simulink model "encode_decode_withAlarms"  (R2022b)
settings: Solver=VariableStepAuto  StartTime=0.0  StopTime=160  RelTol=1e-3
libraries: simulink x8, spsSampleandHoldLib x3
settings Model: Creator=mluser  LastModifiedBy=mluser

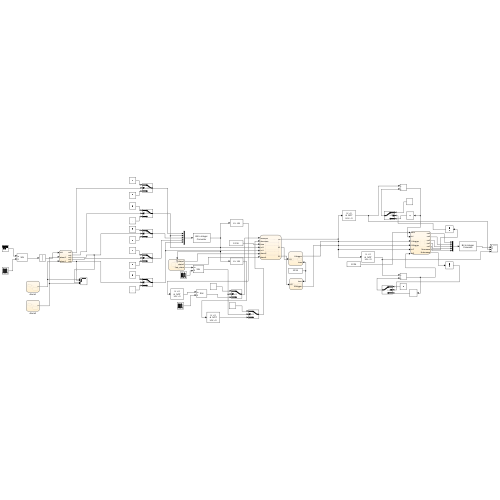
[thumbnail: Simulink's stored preview of the top-level diagram]
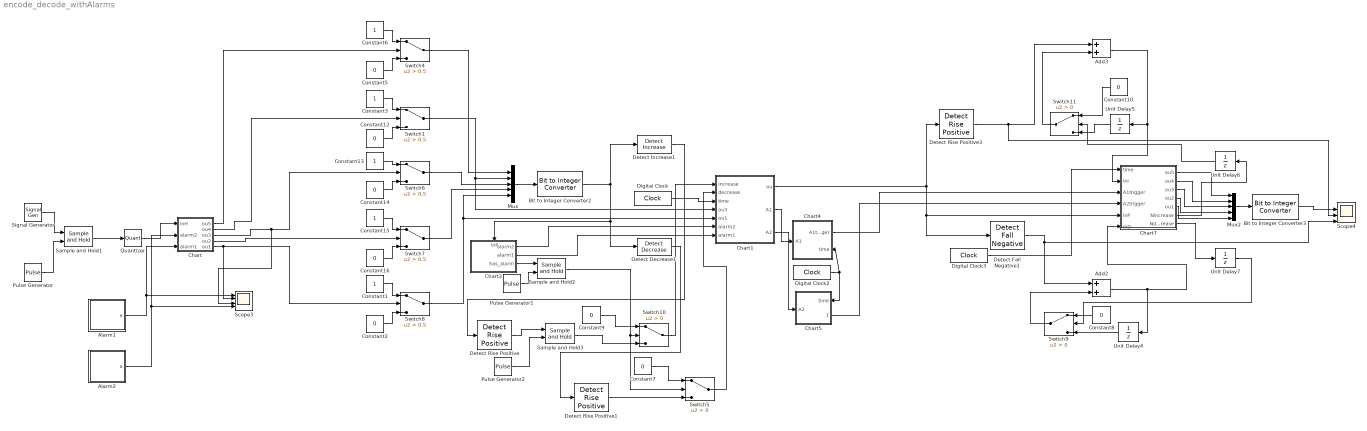
== system encode_decode_withAlarms ==
  Add2 : Sum
  Add3 : Sum
  Alarm1 : Stateflow chart  TreatAsAtomicUnit=on
  Alarm2 : Stateflow chart  TreatAsAtomicUnit=on
  Bit to Integer Converter2 : simulink/Logic and Bit Operations/Bit to Integer Converter  nbits=5  bitOrder=MSB first  signedOutputValues=Unsigned  outDtype=Inherit via internal rule  outDtypeSigned=Inherit via internal rule
      settings: LibrarySourceBlock=|
      | commutil2/Bit to Integer
      | Converter
  Bit to Integer Converter3 : simulink/Logic and Bit Operations/Bit to Integer Converter  nbits=5  bitOrder=MSB first  signedOutputValues=Unsigned  outDtype=Inherit via internal rule  outDtypeSigned=Inherit via internal rule
      settings: LibrarySourceBlock=|
      | commutil2/Bit to Integer
      | Converter
  Chart : Stateflow chart  TreatAsAtomicUnit=on
      settings: PortSchema="{\"entries\":[{\"content\":{\"sides\":[{\"content\":{\"connectorIds\":[\"In1\",\"In2\",\"In3\"]},\"type\":\"ConnectorPlacement.EquallySpacedRectSide\",\"uuid\":\"aaeedc4a-65ef-4d8f-ba01-1ddc4e011816\"},{\"content\":{\"connectorIds\":[\"Out5\",\"Out2\",\"Out1\",\"Out3\",\"Out4\"],\"side\":\"RIGHT\"},\"type\":\"ConnectorPlacement.EquallySpacedRectSide\",\"uuid\":\"bfc75945-f598-4b29-99c0-df6bb3f156b5\"},{\"content\":{\"connectorIds\":[],\"side\":\"TOP\"},\"type\":\"ConnectorPlacement.EquallySpacedRectSide\",\"uuid\":\"e78d9c07-753c-4a5b-aa63-095c584c660c\"}]},\"type\":\"ConnectorPlacement.EquallySpacedConnector\",\"uuid\":\"f46ef6be-e67f-4bb7-838b-d108f8d3e6f5\"}],\"packageUris\":[\"http://schema.mathworks.com/mf0/Connector/R2020b\"],\"version\":\"1.0\"}"
  Chart1 : Stateflow chart  TreatAsAtomicUnit=on
  Chart3 : Stateflow chart  TreatAsAtomicUnit=on
      settings: PortSchema="{\"entries\":[{\"content\":{\"sides\":[{\"content\":{\"connectorIds\":[]},\"type\":\"ConnectorPlacement.EquallySpacedRectSide\",\"uuid\":\"5c3dd9c4-40fc-475e-8fc4-53a3db762fc4\"},{\"content\":{\"connectorIds\":[\"Out1\",\"Out2\",\"Out3\"],\"side\":\"RIGHT\"},\"type\":\"ConnectorPlacement.EquallySpacedRectSide\",\"uuid\":\"288f4f63-e8ff-4ace-a90f-863d45689e1d\"},{\"content\":{\"connectorIds\":[\"In1\"],\"side\":\"TOP\"},\"type\":\"ConnectorPlacement.EquallySpacedRectSide\",\"uuid\":\"c4c1c7c7-df9c-4060-9033-81f7d31c6bbf\"}]},\"type\":\"ConnectorPlacement.EquallySpacedConnector\",\"uuid\":\"fd27b28a-c6e9-46f2-af96-6d8beda93238\"}],\"packageUris\":[\"http://schema.mathworks.com/mf0/Connector/R2020b\"],\"version\":\"1.0\"}"
  Chart4 : Stateflow chart  TreatAsAtomicUnit=on
      settings: PortSchema="{\"entries\":[{\"content\":{\"sides\":[{\"content\":{\"connectorIds\":[\"In2\"]},\"type\":\"ConnectorPlacement.EquallySpacedRectSide\",\"uuid\":\"446bd760-2446-4d27-a1b4-b9f2637686cc\"},{\"content\":{\"connectorIds\":[\"Out1\",\"In1\"],\"side\":\"RIGHT\"},\"type\":\"ConnectorPlacement.EquallySpacedRectSide\",\"uuid\":\"31dc2807-aea3-41af-817a-dc746d332e0b\"},{\"content\":{\"connectorIds\":[],\"side\":\"TOP\"},\"type\":\"ConnectorPlacement.EquallySpacedRectSide\",\"uuid\":\"1029dd63-400c-467c-987d-c8090033263d\"},{\"content\":{\"connectorIds\":[],\"side\":\"BOTTOM\"},\"type\":\"ConnectorPlacement.EquallySpacedRectSide\",\"uuid\":\"3be6e891-aee5-42f4-8a4a-273d783635a4\"}]},\"type\":\"ConnectorPlacement.EquallySpacedConnector\",\"uuid\":\"838269c8-6f3e-4b67-b3d3-f8aaab74d030\"}],\"packageUris\":[\"http://schema.mathworks.com/mf0/Connector/R2020b\"],\"version\":\"1.0\"}"
  Chart5 : Stateflow chart  TreatAsAtomicUnit=on
      settings: PortSchema="{\"entries\":[{\"content\":{\"sides\":[{\"content\":{\"connectorIds\":[\"In2\"]},\"type\":\"ConnectorPlacement.EquallySpacedRectSide\",\"uuid\":\"446bd760-2446-4d27-a1b4-b9f2637686cc\"},{\"content\":{\"connectorIds\":[\"In1\",\"Out1\"],\"side\":\"RIGHT\"},\"type\":\"ConnectorPlacement.EquallySpacedRectSide\",\"uuid\":\"31dc2807-aea3-41af-817a-dc746d332e0b\"},{\"content\":{\"connectorIds\":[],\"side\":\"TOP\"},\"type\":\"ConnectorPlacement.EquallySpacedRectSide\",\"uuid\":\"1029dd63-400c-467c-987d-c8090033263d\"}]},\"type\":\"ConnectorPlacement.EquallySpacedConnector\",\"uuid\":\"838269c8-6f3e-4b67-b3d3-f8aaab74d030\"}],\"packageUris\":[\"http://schema.mathworks.com/mf0/Connector/R2020b\"],\"version\":\"1.0\"}"
  Chart7 : Stateflow chart  TreatAsAtomicUnit=on
      settings: PortSchema="{\"entries\":[{\"content\":{\"sides\":[{\"content\":{\"connectorIds\":[\"In1\",\"In4\",\"In5\",\"In6\",\"In3\",\"In2\"]},\"type\":\"ConnectorPlacement.EquallySpacedRectSide\",\"uuid\":\"2f71a724-cbde-41d0-addd-3c968d2e9507\"},{\"content\":{\"connectorIds\":[\"Out7\",\"Out2\",\"Out3\",\"Out1\",\"Out4\",\"Out5\",\"Out6\"],\"side\":\"RIGHT\"},\"type\":\"ConnectorPlacement.EquallySpacedRectSide\",\"uuid\":\"fd511e75-9748-4994-ae8b-80feb2a63518\"},{\"content\":{\"connectorIds\":[],\"side\":\"TOP\"},\"type\":\"ConnectorPlacement.EquallySpacedRectSide\",\"uuid\":\"1de50c17-1645-4694-9a4a-35d7a7d0bb59\"}]},\"type\":\"ConnectorPlacement.EquallySpacedConnector\",\"uuid\":\"36ccd1b3-f5fe-461c-b238-a087658ad9ff\"}],\"packageUris\":[\"http://schema.mathworks.com/mf0/Connector/R2020b\"],\"version\":\"1.0\"}"
  Constant{1,3,6,13,15} (5 alike) : Constant
  Constant{2,5,7..10,12,14,16} (9 alike) : Constant  Value=0
  Detect Decrease1 : simulink/Logic and Bit Operations/Detect Decrease  vinit=0.0  OutDataTypeStr=boolean
  Detect Increase1 : simulink/Logic and Bit Operations/Detect Increase  vinit=0.0  OutDataTypeStr=boolean
  Detect Fall Negative1 : simulink/Logic and Bit Operations/Detect Fall Negative  vinit=0  OutDataTypeStr=boolean
  Detect Rise Positive : simulink/Logic and Bit Operations/Detect Rise Positive  vinit=0  OutDataTypeStr=boolean
  Detect Rise Positive1 : simulink/Logic and Bit Operations/Detect Rise Positive  vinit=0  OutDataTypeStr=boolean
  Detect Rise Positive3 : simulink/Logic and Bit Operations/Detect Rise Positive  vinit=0  OutDataTypeStr=boolean
  Digital Clock : DigitalClock  SampleTime=0.01
  Digital Clock2 : DigitalClock  SampleTime=0.01
  Digital Clock3 : DigitalClock  SampleTime=0.01
  Mux : Mux  Inputs=5
  Mux2 : Mux  Inputs=5
  Pulse Generator : DiscretePulseGenerator  PulseType=Time based  Period=0.01  PulseWidth=5  PhaseDelay=0.1
  Pulse Generator1 : DiscretePulseGenerator  PulseType=Time based  Period=0.2  PulseWidth=5  PhaseDelay=0.1
  Pulse Generator2 : DiscretePulseGenerator  PulseType=Time based  Period=0.05  PulseWidth=5  PhaseDelay=0.1
  Quantizer : Quantizer
  Sample and Hold1 : spsSampleandHoldLib/Sample and Hold  ic=0  Ts=0.1
      settings: LibrarySourceBlock=|
      | sps_lib/Control/Sample and
      | Hold
  Sample and Hold2 : spsSampleandHoldLib/Sample and Hold  ic=0  Ts=0.1
      settings: LibrarySourceBlock=|
      | sps_lib/Control/Sample and
      | Hold
  Sample and Hold3 : spsSampleandHoldLib/Sample and Hold  ic=0  Ts=0.1
      settings: LibrarySourceBlock=|
      | sps_lib/Control/Sample and
      | Hold
  Scope3 : Scope  NumInputPorts=5
  Scope4 : Scope  NumInputPorts=4
  Signal Generator : SignalGenerator  Amplitude=40  Frequency=0.02  Units=rad/sec
  Switch{1,4,6..8} (5 alike) : Switch  Criteria=u2 > Threshold  Threshold=0.5  SaturateOnIntegerOverflow=off  InputSameDT=off
  Switch{5,9..11} (4 alike) : Switch  Criteria=u2 > Threshold  SaturateOnIntegerOverflow=off  InputSameDT=off
  Unit Delay{4..7} (4 alike) : UnitDelay  SampleTime=-1  HasFrameUpgradeWarning=on
  wires:
  Constant1/1 -> Switch8/1
  Switch1/1 -> Mux/2, Chart1/4(ou3)
  Sample and Hold1/1 -> Quantizer/1
  Chart/3(ou2) -> Switch7/2
  Constant14/1 -> Switch6/3
  Mux/1 -> Bit to Integer Converter2/1
  Digital Clock/1 -> Chart1/3(time)
  Pulse Generator/1 -> Sample and Hold1/2
  Constant2/1 -> Switch8/3
  Constant13/1 -> Switch6/1
  Chart/5(ou5) -> Switch4/2
  Constant6/1 -> Switch4/1
  Chart/2(ou4) -> Switch1/2
  Constant15/1 -> Switch7/1
  Bit to Integer Converter2/1 -> Chart3/1(inP), Detect Decrease1/1, Detect Increase1/1
  Signal Generator/1 -> Sample and Hold1/1
  Constant3/1 -> Switch1/1
  Constant12/1 -> Switch1/3
  Quantizer/1 -> Chart/1(inH)
  Constant5/1 -> Switch4/3
  Constant16/1 -> Switch7/3
  Switch8/1 -> Mux/5, Chart1/5(ou1)
  Chart/4(ou1) -> Switch8/2, Scope3/2
  Alarm2/1(a) -> Scope3/5, Chart/2(alarm2)
  Switch6/1 -> Mux/3
  Chart/1(ou3) -> Scope3/4, Switch6/2
  Switch4/1 -> Mux/1
  Switch7/1 -> Mux/4
  Alarm1/1(a) -> Scope3/1, Chart/3(alarm1)
  Detect Decrease1/1 -> Detect Rise Positive1/1
  Switch10/1 -> Chart1/1(increase)
  Detect Rise Positive1/1 -> Switch5/3
  Constant7/1 -> Switch5/1
  Switch5/1 -> Chart1/2(decrease)
  Sample and Hold2/1 -> Switch5/2, Switch10/2
  Chart3/3(has_alarm) -> Sample and Hold2/1
  Pulse Generator1/1 -> Sample and Hold2/2
  Chart3/2(alarm1) -> Chart1/7(alarm1)
  Chart3/1(alarm2) -> Chart1/6(alarm2)
  Detect Increase1/1 -> Detect Rise Positive/1
  Detect Rise Positive/1 -> Sample and Hold3/1
  Pulse Generator2/1 -> Sample and Hold3/2
  Sample and Hold3/1 -> Switch10/3
  Constant9/1 -> Switch10/1
  Chart1/2(A1) -> Chart4/2(A1)
  Chart1/3(A2) -> Chart5/2(A2)
  Switch9/1 -> Add2/2
  Unit Delay6/1 -> Switch11/2
  Add3/1 -> Chart7/4(inI), Unit Delay5/1
  Chart7/5(Nincrease) -> Unit Delay6/1
  Unit Delay5/1 -> Switch11/3
  Unit Delay7/1 -> Switch9/2
  Add2/1 -> Chart7/2(inD), Unit Delay4/1
  Switch11/1 -> Add3/2
  Detect Fall Negative1/1 -> Scope4/4, Add2/1
  Constant8/1 -> Switch9/1
  Chart7/3(ou3) -> Mux2/3
  Constant10/1 -> Switch11/1
  Chart7/1(ou2) -> Mux2/4
  Digital Clock3/1 -> Chart7/1(time)
  Chart7/2(ou4) -> Mux2/2
  Unit Delay4/1 -> Switch9/3
  Mux2/1 -> Bit to Integer Converter3/1
  Chart7/7(ou5) -> Mux2/1
  Chart1/1(ou) -> Chart7/3(inP), Detect Fall Negative1/1, Detect Rise Positive3/1
  Chart7/6(Ndecrease) -> Unit Delay7/1
  Bit to Integer Converter3/1 -> Scope4/2
  Detect Rise Positive3/1 -> Scope4/3, Add3/1
  Chart7/4(ou1) -> Mux2/5
  Digital Clock2/1 -> Chart5/1(time), Chart4/1(time)
  Chart4/1(A1trigger) -> Chart7/5(A1trigger)
  Chart5/1(A2trigger) -> Chart7/6(A2trigger)

== stateflow chart encode_decode_withAlarms/Chart1 ==
  (junction 100) -> (junction 140) [order 2] : [alarm1==1]
  (junction 140) -> (junction 131) : {A1=1;}
  (default) -> (junction 100) : {A1=0;A2=0;}
  (junction 100) -> (junction 95) [order 1]
  (junction 131) -> (junction 128)
  (junction 134) -> (junction 128) : {A2=1;}
  (junction 95) -> (junction 134) [order 2] : [alarm2==1]
  (junction 128) -> (junction 44)
  (junction 95) -> (junction 3) [order 1]
  (junction 3) -> (junction 28) [order 2] : [increase==1&&time>0]
  (junction 28) -> (junction 44) : {ou=1;}
  (junction 3) -> (junction 10) [order 1]
  (junction 44) -> (junction 43)
  (junction 10) -> (junction 8) [order 1] : [decrease==1&&time>0]
  (junction 8) -> (junction 43) : {ou=-1;}
  (junction 10) -> (junction 71) [order 2]
  (junction 43) -> (junction 72)
  (junction 71) -> (junction 73) [order 1] : [time==0&&ou3==1]
  (junction 73) -> (junction 72) : {ou=1;}
  (junction 71) -> (junction 78) [order 2]
  (junction 72) -> (junction 80)
  (junction 78) -> (junction 79) [order 1] : [time==0&&ou1==0]
  (junction 79) -> (junction 80) : {ou=-1;}
  (junction 78) -> (junction 90) [order 2]
  (junction 80) -> (junction 88)
  (junction 89) -> (junction 88) : {ou=0}
  (junction 90) -> (junction 89) : [increase==0&&decrease==0]
  data: increase input; decrease input; ou output; time input; ou3 input; ou1 input; alarm2 input; A1 output; A2 output; alarm1 input

== stateflow chart encode_decode_withAlarms/Chart ==
  (default) -> (junction 100) : {ou1=0;
      | ou2=0;
      | ou3=0;
      | ou4=0;
      | ou5=0;
      | }
  (junction 100) -> (junction 101) [order 1] : [alarm1==1]
  (junction 101) -> (junction 102) : {ou1=1;ou2=1;ou3=1;ou4=1;ou5=1;}
  (junction 100) -> (junction 103) [order 2]
  (junction 102) -> (junction 105)
  (junction 103) -> (junction 104) [order 1] : [alarm2==1]
  (junction 104) -> (junction 105) : {ou1=0;ou2=1;ou3=1;ou4=1;ou5=1;}
  (junction 103) -> (junction 3) [order 2]
  (junction 105) -> (junction 44)
  (junction 3) -> (junction 28) [order 2] : [inH==0]
  (junction 28) -> (junction 44) : {ou1=0;ou2=0;ou3=0;ou4=0;}
  (junction 3) -> (junction 10) [order 1]
  (junction 44) -> (junction 43)
  (junction 10) -> (junction 8) [order 1] : [inH<=10]
  (junction 8) -> (junction 43) : {ou1=1;ou2=0;ou3=0;ou4=0;ou5=0}
  (junction 10) -> (junction 12) [order 2]
  (junction 43) -> (junction 42)
  (junction 16) -> (junction 42) : {ou1=1;ou2=1;ou3=0;ou4=0;ou5=0;}
  (junction 12) -> (junction 16) [order 1] : [inH>10&&inH<=20]
  (junction 42) -> (junction 41)
  (junction 12) -> (junction 19) [order 2]
  (junction 19) -> (junction 18) [order 1] : [inH>20&&inH<=30]
  (junction 18) -> (junction 41) : {ou1=1;ou2=1;ou3=1;ou4=0;ou5=0;}
  (junction 41) -> (junction 63)
  (junction 19) -> (junction 61) [order 2]
  (junction 61) -> (junction 62) : [inH>30]
  (junction 62) -> (junction 63) : {ou1=1;ou2=1;ou3=1;ou4=1;ou5=0;}
  data: ou3 output; ou4 output; ou2 output; ou1 output; inH input; alarm2 input; alarm1 input; ou5 output

== stateflow chart encode_decode_withAlarms/Chart3 ==
  state alarm1
    entry:
    alarm1=1;
    has_alarm=1;
    after(0.2,sec);
  state alarm_detect
    entry:
    alarm1=0;
    alarm2=0;
    has_alarm=0;
  state alarm2
    entry:
    alarm2=1;
    has_alarm=1;
    after(0.2,sec);
  alarm_detect -> alarm1 [order 1] : [inP==31]
  (default) -> alarm_detect
  alarm1 -> alarm_detect : [inP<20]
  alarm_detect -> alarm2 [order 2] : [inP==30]
  alarm2 -> alarm_detect : [inP<20]
  data: inP input; alarm2 output; alarm1 output; has_alarm output

== stateflow chart encode_decode_withAlarms/Chart4 ==
  state begin
    entry:
    A1trigger=0;
    A1time=0;
  state end
    entry:
    A1trigger=1;
    A1time=time;
  (default) -> begin : {A1trigger=0;}
  begin -> end : [A1==1]
  end -> begin : [A1==0]
  data: time input; A1trigger output; A1 input

== stateflow chart encode_decode_withAlarms/Alarm1 ==
  state begin
    du:a=0;
  state end
    du:a=1;
  (default) -> begin
  begin -> end : after(100,sec)
  end -> begin : after(0.2,sec)
  data: a output

== stateflow chart encode_decode_withAlarms/Alarm2 ==
  state begin
    du:a=0;
  state end
    du:a=1;
  (default) -> begin
  begin -> end : after(70,sec)
  end -> begin : after(0.2,sec)
  data: a output

== stateflow chart encode_decode_withAlarms/Chart5 ==
  state begin
    entry:
    A2trigger=0;
    A2time=0;
  state end
    entry:
    A2trigger=1;
    A2time=time;
  (default) -> begin : {A2trigger=0;}
  begin -> end : [A2==1]
  end -> begin : [A2==0]
  data: time input; A2trigger output; A2 input

== stateflow chart encode_decode_withAlarms/Chart7 ==
  state Decoder
    entry:
    state Normal_water_level_measure
      entry:
      state state1
        entry:
        ou1=0;ou2=0;
        ou3=0;ou4=0;
        ou5=0;
        Ndecrease=0;
        Nincrease=0;
      state initial
        entry:
        Ndecrease=0;
        Nincrease=0;
      state state2
        entry:
        ou1=1;ou2=0;
        ou3=0;ou4=0;
        ou5=0;
        Ndecrease=0;
        Nincrease=0;
      state state3
        entry:
        ou1=1;ou2=1;
        ou3=0;ou4=0;ou5=0
        Ndecrease=0;
        Nincrease=0;
      state state5
        entry:
        ou1=1;ou2=1;
        ou3=1;ou4=1;ou5=0;
        Ndecrease=0;
        Nincrease=0;
      state state4
        entry:
        ou1=1;ou2=1;
        ou3=1;ou4=0;ou5=0;
        Nincrease=0;
        Ndecrease=0;
      (default) -> initial
      state1 -> state2 : [time>=1&&inP==1&&inI==1]
      initial -> state1 [order 2] : [time<1&&inP==1]
          | {Ndecrease=0;
          | Nincrease=0;}
      (junction 120) -> state1 : {Ndecrease=1;
          | Nincrease=1;}
      initial -> state5 [order 1] : [time<1&&inP==-1]
      state2 -> (junction 120) [order 2] : [time>=1&&inP==-1&&inD==3]
      state3 -> state2 [order 2] : [time>=1&&inP==-1&&inD==3]
      state2 -> state3 [order 1] : [time>=1&&inP==1&&inI==1]
      state4 -> state3 [order 2] : [time>=1&&inP==-1&&inD==2]
      state3 -> state4 [order 1] : [time>=1&&inP==1&&inI==2]
      state4 -> (junction 124) [order 1] : [time>=1&&inP==1&&inI==2]
      (junction 124) -> state5 : {Ndecrease=1;
          | Nincrease=1;}
      state5 -> state4 : [time>=1&&inP==-1&&inD==1]
    state Alarm_triggering
      entry:
      state ALarm1
        entry:
        ou1=1;ou2=1;
        ou3=1;ou4=1;ou5=1;
        Ndecrease=0;
        Nincrease=0;
      state Alarm2
        entry:
        ou1=0;ou2=1;
        ou3=1;ou4=1;ou5=1;
        Ndecrease=0;
        Nincrease=0;
      (default) -> ALarm1
      Alarm2 -> ALarm1 : [A1trigger==1]
      ALarm1 -> Alarm2 : [A2trigger==1]
    (default) -> Normal_water_level_measure
    Normal_water_level_measure -> Alarm_triggering : [A1trigger==1||A2trigger==1]
        | {Ndecrease=1;Nincrease=1;}
    Alarm_triggering -> Normal_water_level_measure : [A1trigger==0&&A2trigger==0]
        | {Nincrease=1;Ndecrease=1;}
  (default) -> Decoder : {ou1=0;ou2=0;
      | ou3=0;ou4=0;ou5=0;}
  data: time input; inD input; inP input; inI input; ou2 output; ou4 output; ou3 output; ou1 output; Nincrease output; Ndecrease output; A1trigger input; A2trigger input; ou5 output
